simulink model "soc_dvbs2_fpga"  (R2025b)
settings: Solver=FixedStepDiscrete  StartTime=0.0  StopTime=0  RelTol=1e-3
InitFcn:
  | soc_dvbs2_init;
values from neighbouring files (symbols this model uses):
  Rsym = 4e6    (= 4000000)    [soc_dvbs2_init.m]
  soc_dvbs2_txPacketBits = [1 1 0 1 0 1 1 1 0 1 1 1 ... (2972 elements, 2972x1)]    [soc_dvbs2_txPacketBits.mat]
  syncWord = (dec2bin(hex2dec('AC')) - '0').'    [soc_dvbs2_init.m]
  txDataOut = txobj(frameBits(:))    [soc_dvbs2_init.m]
  txFiltCoeff = txobj.pTxFilterCoeff    [soc_dvbs2_init.m]
undefined symbols (not defined in the file or in its folder): Add, coefficientsLog, coefficientsSqrt1, coefficientsSqrt2, dataBits, designMultirateFIR, noisePow, NumBits1, NumBits2, seedsURNG1, seedsURNG2, Shift, Slope1, Slope2, soc_dvbs2_designFIRFilter, txDataOutS1, txDataOutS10, txDataOutS12, txDataOutS13, txDataOutS14, txDataOutS15, txDataOutS16, txDataOutS18, txDataOutS19, txDataOutS2, txDataOutS20, txDataOutS21, txDataOutS22, txDataOutS24, txDataOutS25, txDataOutS26, txDataOutS27, txDataOutS3, txDataOutS4, txDataOutS5, txDataOutS6, txDataOutS7, txDataOutS8, txDataOutS9
libraries: simulink x214, hdlsllib x211, dspsigops x22, dsphdlfiltering2 x8, dsphdlsigops2 x5, commseqgen3 x5, dsphdlmathfun2 x3, hwlogicconnlib x2, whdledac x2, commhdlcrc x2, whdlutilities x1, whdlmod x1
(part 5 of 12)

== system soc_dvbs2_fpga/DVBS2/DVBS2 TxRx/LUT Based Tx/Subsystem1/Subsystem1/txLUT5 ==
  rst : Inport
  enb : Inport  Port=2
  1-D Lookup Table : Lookup_n-D  NumberOfTableDimensions=1  BreakpointsSpecification=Even spacing  BreakpointsForDimension1=0:length(txDataOut)-1  BreakpointsForDimension1FirstPoint=0  Table=fi(DataLUT,1,18,16)  TableDataTypeStr=Inherit: Inherit from 'Table data'  InterpMethod=Flat  InternalRulePriority=Speed  OutDataTypeStr=Inherit: Inherit from 'Table data'  RndMeth=Simplest
  Compare To Constant : simulink/Logic and Bit Operations/Compare To Constant  relop===  const=length(DataLUT) - 2  OutDataTypeStr=boolean
  HDL Counter : hdlsllib/Sources/HDL Counter  CountType=Count limited  CountInit=0  CountStep=1  CountMax=length(DataLUT)-1  CountFromType=Initial value  CountFrom=0  CountResetPort=on  CountLoadPort=off  CountEnbPort=on  CountDirPort=off  CountHitOutputPort=off  CountDataType=Unsigned  CountWordLen=nextpow2(length(DataLUT)-1)  CountFracLen=0  CountSampTime=1
  Out1 : Outport
  endOfLUT : Outport  Port=2
  wires:
  1-D Lookup Table/1 -> Out1/1
  HDL Counter/1 -> Compare To Constant/1, 1-D Lookup Table/1
  enb/1 -> HDL Counter/2
  Compare To Constant/1 -> endOfLUT/1
  rst/1 -> HDL Counter/1

== system soc_dvbs2_fpga/DVBS2/DVBS2 TxRx/LUT Based Tx/Subsystem1/Subsystem1/txLUT6 ==
  rst : Inport
  enb : Inport  Port=2
  1-D Lookup Table : Lookup_n-D  NumberOfTableDimensions=1  BreakpointsSpecification=Even spacing  BreakpointsForDimension1=0:length(txDataOut)-1  BreakpointsForDimension1FirstPoint=0  Table=fi(DataLUT,1,18,16)  TableDataTypeStr=Inherit: Inherit from 'Table data'  InterpMethod=Flat  InternalRulePriority=Speed  OutDataTypeStr=Inherit: Inherit from 'Table data'  RndMeth=Simplest
  Compare To Constant : simulink/Logic and Bit Operations/Compare To Constant  relop===  const=length(DataLUT) - 2  OutDataTypeStr=boolean
  HDL Counter : hdlsllib/Sources/HDL Counter  CountType=Count limited  CountInit=0  CountStep=1  CountMax=length(DataLUT)-1  CountFromType=Initial value  CountFrom=0  CountResetPort=on  CountLoadPort=off  CountEnbPort=on  CountDirPort=off  CountHitOutputPort=off  CountDataType=Unsigned  CountWordLen=nextpow2(length(DataLUT)-1)  CountFracLen=0  CountSampTime=1
  Out1 : Outport
  endOfLUT : Outport  Port=2
  wires:
  rst/1 -> HDL Counter/1
  Compare To Constant/1 -> endOfLUT/1
  enb/1 -> HDL Counter/2
  HDL Counter/1 -> 1-D Lookup Table/1, Compare To Constant/1
  1-D Lookup Table/1 -> Out1/1

== system soc_dvbs2_fpga/DVBS2/DVBS2 TxRx/LUT Based Tx/Subsystem1/Subsystem2/txLUT1 ==
  rst : Inport
  enb : Inport  Port=2
  1-D Lookup Table : Lookup_n-D  NumberOfTableDimensions=1  BreakpointsSpecification=Even spacing  BreakpointsForDimension1=0:length(txDataOut)-1  BreakpointsForDimension1FirstPoint=0  Table=fi(DataLUT,1,18,16)  TableDataTypeStr=Inherit: Inherit from 'Table data'  InterpMethod=Flat  InternalRulePriority=Speed  OutDataTypeStr=Inherit: Inherit from 'Table data'  RndMeth=Simplest
  Compare To Constant : simulink/Logic and Bit Operations/Compare To Constant  relop===  const=length(DataLUT) - 2  OutDataTypeStr=boolean
  HDL Counter : hdlsllib/Sources/HDL Counter  CountType=Count limited  CountInit=0  CountStep=1  CountMax=length(DataLUT)-1  CountFromType=Initial value  CountFrom=0  CountResetPort=on  CountLoadPort=off  CountEnbPort=on  CountDirPort=off  CountHitOutputPort=off  CountDataType=Unsigned  CountWordLen=nextpow2(length(DataLUT)-1)  CountFracLen=0  CountSampTime=1
  Out1 : Outport
  endOfLUT : Outport  Port=2
  wires:
  rst/1 -> HDL Counter/1
  Compare To Constant/1 -> endOfLUT/1
  enb/1 -> HDL Counter/2
  HDL Counter/1 -> 1-D Lookup Table/1, Compare To Constant/1
  1-D Lookup Table/1 -> Out1/1

== system soc_dvbs2_fpga/DVBS2/DVBS2 TxRx/LUT Based Tx/Subsystem1/Subsystem2/txLUT2 ==
  rst : Inport
  enb : Inport  Port=2
  1-D Lookup Table : Lookup_n-D  NumberOfTableDimensions=1  BreakpointsSpecification=Even spacing  BreakpointsForDimension1=0:length(txDataOut)-1  BreakpointsForDimension1FirstPoint=0  Table=fi(DataLUT,1,18,16)  TableDataTypeStr=Inherit: Inherit from 'Table data'  InterpMethod=Flat  InternalRulePriority=Speed  OutDataTypeStr=Inherit: Inherit from 'Table data'  RndMeth=Simplest
  Compare To Constant : simulink/Logic and Bit Operations/Compare To Constant  relop===  const=length(DataLUT) - 2  OutDataTypeStr=boolean
  HDL Counter : hdlsllib/Sources/HDL Counter  CountType=Count limited  CountInit=0  CountStep=1  CountMax=length(DataLUT)-1  CountFromType=Initial value  CountFrom=0  CountResetPort=on  CountLoadPort=off  CountEnbPort=on  CountDirPort=off  CountHitOutputPort=off  CountDataType=Unsigned  CountWordLen=nextpow2(length(DataLUT)-1)  CountFracLen=0  CountSampTime=1
  Out1 : Outport
  endOfLUT : Outport  Port=2
  wires:
  1-D Lookup Table/1 -> Out1/1
  HDL Counter/1 -> Compare To Constant/1, 1-D Lookup Table/1
  enb/1 -> HDL Counter/2
  Compare To Constant/1 -> endOfLUT/1
  rst/1 -> HDL Counter/1

== system soc_dvbs2_fpga/DVBS2/DVBS2 TxRx/LUT Based Tx/Subsystem1/Subsystem2/txLUT3 ==
  rst : Inport
  enb : Inport  Port=2
  1-D Lookup Table : Lookup_n-D  NumberOfTableDimensions=1  BreakpointsSpecification=Even spacing  BreakpointsForDimension1=0:length(txDataOut)-1  BreakpointsForDimension1FirstPoint=0  Table=fi(DataLUT,1,18,16)  TableDataTypeStr=Inherit: Inherit from 'Table data'  InterpMethod=Flat  InternalRulePriority=Speed  OutDataTypeStr=Inherit: Inherit from 'Table data'  RndMeth=Simplest
  Compare To Constant : simulink/Logic and Bit Operations/Compare To Constant  relop===  const=length(DataLUT) - 2  OutDataTypeStr=boolean
  HDL Counter : hdlsllib/Sources/HDL Counter  CountType=Count limited  CountInit=0  CountStep=1  CountMax=length(DataLUT)-1  CountFromType=Initial value  CountFrom=0  CountResetPort=on  CountLoadPort=off  CountEnbPort=on  CountDirPort=off  CountHitOutputPort=off  CountDataType=Unsigned  CountWordLen=nextpow2(length(DataLUT)-1)  CountFracLen=0  CountSampTime=1
  Out1 : Outport
  endOfLUT : Outport  Port=2
  wires:
  1-D Lookup Table/1 -> Out1/1
  HDL Counter/1 -> Compare To Constant/1, 1-D Lookup Table/1
  enb/1 -> HDL Counter/2
  Compare To Constant/1 -> endOfLUT/1
  rst/1 -> HDL Counter/1

== system soc_dvbs2_fpga/DVBS2/DVBS2 TxRx/LUT Based Tx/Subsystem1/Subsystem2/txLUT4 ==
  rst : Inport
  enb : Inport  Port=2
  1-D Lookup Table : Lookup_n-D  NumberOfTableDimensions=1  BreakpointsSpecification=Even spacing  BreakpointsForDimension1=0:length(txDataOut)-1  BreakpointsForDimension1FirstPoint=0  Table=fi(DataLUT,1,18,16)  TableDataTypeStr=Inherit: Inherit from 'Table data'  InterpMethod=Flat  InternalRulePriority=Speed  OutDataTypeStr=Inherit: Inherit from 'Table data'  RndMeth=Simplest
  Compare To Constant : simulink/Logic and Bit Operations/Compare To Constant  relop===  const=length(DataLUT) - 2  OutDataTypeStr=boolean
  HDL Counter : hdlsllib/Sources/HDL Counter  CountType=Count limited  CountInit=0  CountStep=1  CountMax=length(DataLUT)-1  CountFromType=Initial value  CountFrom=0  CountResetPort=on  CountLoadPort=off  CountEnbPort=on  CountDirPort=off  CountHitOutputPort=off  CountDataType=Unsigned  CountWordLen=nextpow2(length(DataLUT)-1)  CountFracLen=0  CountSampTime=1
  Out1 : Outport
  endOfLUT : Outport  Port=2
  wires:
  rst/1 -> HDL Counter/1
  Compare To Constant/1 -> endOfLUT/1
  enb/1 -> HDL Counter/2
  HDL Counter/1 -> 1-D Lookup Table/1, Compare To Constant/1
  1-D Lookup Table/1 -> Out1/1

== system soc_dvbs2_fpga/DVBS2/DVBS2 TxRx/LUT Based Tx/Subsystem1/Subsystem2/txLUT5 ==
  rst : Inport
  enb : Inport  Port=2
  1-D Lookup Table : Lookup_n-D  NumberOfTableDimensions=1  BreakpointsSpecification=Even spacing  BreakpointsForDimension1=0:length(txDataOut)-1  BreakpointsForDimension1FirstPoint=0  Table=fi(DataLUT,1,18,16)  TableDataTypeStr=Inherit: Inherit from 'Table data'  InterpMethod=Flat  InternalRulePriority=Speed  OutDataTypeStr=Inherit: Inherit from 'Table data'  RndMeth=Simplest
  Compare To Constant : simulink/Logic and Bit Operations/Compare To Constant  relop===  const=length(DataLUT) - 2  OutDataTypeStr=boolean
  HDL Counter : hdlsllib/Sources/HDL Counter  CountType=Count limited  CountInit=0  CountStep=1  CountMax=length(DataLUT)-1  CountFromType=Initial value  CountFrom=0  CountResetPort=on  CountLoadPort=off  CountEnbPort=on  CountDirPort=off  CountHitOutputPort=off  CountDataType=Unsigned  CountWordLen=nextpow2(length(DataLUT)-1)  CountFracLen=0  CountSampTime=1
  Out1 : Outport
  endOfLUT : Outport  Port=2
  wires:
  1-D Lookup Table/1 -> Out1/1
  HDL Counter/1 -> Compare To Constant/1, 1-D Lookup Table/1
  enb/1 -> HDL Counter/2
  Compare To Constant/1 -> endOfLUT/1
  rst/1 -> HDL Counter/1

== system soc_dvbs2_fpga/DVBS2/DVBS2 TxRx/LUT Based Tx/Subsystem1/Subsystem2/txLUT6 ==
  rst : Inport
  enb : Inport  Port=2
  1-D Lookup Table : Lookup_n-D  NumberOfTableDimensions=1  BreakpointsSpecification=Even spacing  BreakpointsForDimension1=0:length(txDataOut)-1  BreakpointsForDimension1FirstPoint=0  Table=fi(DataLUT,1,18,16)  TableDataTypeStr=Inherit: Inherit from 'Table data'  InterpMethod=Flat  InternalRulePriority=Speed  OutDataTypeStr=Inherit: Inherit from 'Table data'  RndMeth=Simplest
  Compare To Constant : simulink/Logic and Bit Operations/Compare To Constant  relop===  const=length(DataLUT) - 2  OutDataTypeStr=boolean
  HDL Counter : hdlsllib/Sources/HDL Counter  CountType=Count limited  CountInit=0  CountStep=1  CountMax=length(DataLUT)-1  CountFromType=Initial value  CountFrom=0  CountResetPort=on  CountLoadPort=off  CountEnbPort=on  CountDirPort=off  CountHitOutputPort=off  CountDataType=Unsigned  CountWordLen=nextpow2(length(DataLUT)-1)  CountFracLen=0  CountSampTime=1
  Out1 : Outport
  endOfLUT : Outport  Port=2
  wires:
  rst/1 -> HDL Counter/1
  Compare To Constant/1 -> endOfLUT/1
  enb/1 -> HDL Counter/2
  HDL Counter/1 -> 1-D Lookup Table/1, Compare To Constant/1
  1-D Lookup Table/1 -> Out1/1

== system soc_dvbs2_fpga/DVBS2/DVBS2 TxRx/LUT Based Tx/Subsystem1/Subsystem4/txLUT1 ==
  rst : Inport
  enb : Inport  Port=2
  1-D Lookup Table : Lookup_n-D  NumberOfTableDimensions=1  BreakpointsSpecification=Even spacing  BreakpointsForDimension1=0:length(txDataOut)-1  BreakpointsForDimension1FirstPoint=0  Table=fi(DataLUT,1,18,16)  TableDataTypeStr=Inherit: Inherit from 'Table data'  InterpMethod=Flat  InternalRulePriority=Speed  OutDataTypeStr=Inherit: Inherit from 'Table data'  RndMeth=Simplest
  Compare To Constant : simulink/Logic and Bit Operations/Compare To Constant  relop===  const=length(DataLUT) - 2  OutDataTypeStr=boolean
  HDL Counter : hdlsllib/Sources/HDL Counter  CountType=Count limited  CountInit=0  CountStep=1  CountMax=length(DataLUT)-1  CountFromType=Initial value  CountFrom=0  CountResetPort=on  CountLoadPort=off  CountEnbPort=on  CountDirPort=off  CountHitOutputPort=off  CountDataType=Unsigned  CountWordLen=nextpow2(length(DataLUT)-1)  CountFracLen=0  CountSampTime=1
  Out1 : Outport
  endOfLUT : Outport  Port=2
  wires:
  1-D Lookup Table/1 -> Out1/1
  HDL Counter/1 -> Compare To Constant/1, 1-D Lookup Table/1
  enb/1 -> HDL Counter/2
  Compare To Constant/1 -> endOfLUT/1
  rst/1 -> HDL Counter/1

== system soc_dvbs2_fpga/DVBS2/DVBS2 TxRx/LUT Based Tx/Subsystem1/Subsystem4/txLUT2 ==
  rst : Inport
  enb : Inport  Port=2
  1-D Lookup Table : Lookup_n-D  NumberOfTableDimensions=1  BreakpointsSpecification=Even spacing  BreakpointsForDimension1=0:length(txDataOut)-1  BreakpointsForDimension1FirstPoint=0  Table=fi(DataLUT,1,18,16)  TableDataTypeStr=Inherit: Inherit from 'Table data'  InterpMethod=Flat  InternalRulePriority=Speed  OutDataTypeStr=Inherit: Inherit from 'Table data'  RndMeth=Simplest
  Compare To Constant : simulink/Logic and Bit Operations/Compare To Constant  relop===  const=length(DataLUT) - 2  OutDataTypeStr=boolean
  HDL Counter : hdlsllib/Sources/HDL Counter  CountType=Count limited  CountInit=0  CountStep=1  CountMax=length(DataLUT)-1  CountFromType=Initial value  CountFrom=0  CountResetPort=on  CountLoadPort=off  CountEnbPort=on  CountDirPort=off  CountHitOutputPort=off  CountDataType=Unsigned  CountWordLen=nextpow2(length(DataLUT)-1)  CountFracLen=0  CountSampTime=1
  Out1 : Outport
  endOfLUT : Outport  Port=2
  wires:
  rst/1 -> HDL Counter/1
  Compare To Constant/1 -> endOfLUT/1
  enb/1 -> HDL Counter/2
  HDL Counter/1 -> 1-D Lookup Table/1, Compare To Constant/1
  1-D Lookup Table/1 -> Out1/1

== system soc_dvbs2_fpga/DVBS2/DVBS2 TxRx/LUT Based Tx/Subsystem1/Subsystem4/txLUT3 ==
  rst : Inport
  enb : Inport  Port=2
  1-D Lookup Table : Lookup_n-D  NumberOfTableDimensions=1  BreakpointsSpecification=Even spacing  BreakpointsForDimension1=0:length(txDataOut)-1  BreakpointsForDimension1FirstPoint=0  Table=fi(DataLUT,1,18,16)  TableDataTypeStr=Inherit: Inherit from 'Table data'  InterpMethod=Flat  InternalRulePriority=Speed  OutDataTypeStr=Inherit: Inherit from 'Table data'  RndMeth=Simplest
  Compare To Constant : simulink/Logic and Bit Operations/Compare To Constant  relop===  const=length(DataLUT) - 2  OutDataTypeStr=boolean
  HDL Counter : hdlsllib/Sources/HDL Counter  CountType=Count limited  CountInit=0  CountStep=1  CountMax=length(DataLUT)-1  CountFromType=Initial value  CountFrom=0  CountResetPort=on  CountLoadPort=off  CountEnbPort=on  CountDirPort=off  CountHitOutputPort=off  CountDataType=Unsigned  CountWordLen=nextpow2(length(DataLUT)-1)  CountFracLen=0  CountSampTime=1
  Out1 : Outport
  endOfLUT : Outport  Port=2
  wires:
  rst/1 -> HDL Counter/1
  Compare To Constant/1 -> endOfLUT/1
  enb/1 -> HDL Counter/2
  HDL Counter/1 -> 1-D Lookup Table/1, Compare To Constant/1
  1-D Lookup Table/1 -> Out1/1

== system soc_dvbs2_fpga/DVBS2/DVBS2 TxRx/LUT Based Tx/Subsystem1/Subsystem4/txLUT4 ==
  rst : Inport
  enb : Inport  Port=2
  1-D Lookup Table : Lookup_n-D  NumberOfTableDimensions=1  BreakpointsSpecification=Even spacing  BreakpointsForDimension1=0:length(txDataOut)-1  BreakpointsForDimension1FirstPoint=0  Table=fi(DataLUT,1,18,16)  TableDataTypeStr=Inherit: Inherit from 'Table data'  InterpMethod=Flat  InternalRulePriority=Speed  OutDataTypeStr=Inherit: Inherit from 'Table data'  RndMeth=Simplest
  Compare To Constant : simulink/Logic and Bit Operations/Compare To Constant  relop===  const=length(DataLUT) - 2  OutDataTypeStr=boolean
  HDL Counter : hdlsllib/Sources/HDL Counter  CountType=Count limited  CountInit=0  CountStep=1  CountMax=length(DataLUT)-1  CountFromType=Initial value  CountFrom=0  CountResetPort=on  CountLoadPort=off  CountEnbPort=on  CountDirPort=off  CountHitOutputPort=off  CountDataType=Unsigned  CountWordLen=nextpow2(length(DataLUT)-1)  CountFracLen=0  CountSampTime=1
  Out1 : Outport
  endOfLUT : Outport  Port=2
  wires:
  1-D Lookup Table/1 -> Out1/1
  HDL Counter/1 -> Compare To Constant/1, 1-D Lookup Table/1
  enb/1 -> HDL Counter/2
  Compare To Constant/1 -> endOfLUT/1
  rst/1 -> HDL Counter/1

== system soc_dvbs2_fpga/DVBS2/DVBS2 TxRx/LUT Based Tx/Subsystem1/Subsystem4/txLUT5 ==
  rst : Inport
  enb : Inport  Port=2
  1-D Lookup Table : Lookup_n-D  NumberOfTableDimensions=1  BreakpointsSpecification=Even spacing  BreakpointsForDimension1=0:length(txDataOut)-1  BreakpointsForDimension1FirstPoint=0  Table=fi(DataLUT,1,18,16)  TableDataTypeStr=Inherit: Inherit from 'Table data'  InterpMethod=Flat  InternalRulePriority=Speed  OutDataTypeStr=Inherit: Inherit from 'Table data'  RndMeth=Simplest
  Compare To Constant : simulink/Logic and Bit Operations/Compare To Constant  relop===  const=length(DataLUT) - 2  OutDataTypeStr=boolean
  HDL Counter : hdlsllib/Sources/HDL Counter  CountType=Count limited  CountInit=0  CountStep=1  CountMax=length(DataLUT)-1  CountFromType=Initial value  CountFrom=0  CountResetPort=on  CountLoadPort=off  CountEnbPort=on  CountDirPort=off  CountHitOutputPort=off  CountDataType=Unsigned  CountWordLen=nextpow2(length(DataLUT)-1)  CountFracLen=0  CountSampTime=1
  Out1 : Outport
  endOfLUT : Outport  Port=2
  wires:
  rst/1 -> HDL Counter/1
  Compare To Constant/1 -> endOfLUT/1
  enb/1 -> HDL Counter/2
  HDL Counter/1 -> 1-D Lookup Table/1, Compare To Constant/1
  1-D Lookup Table/1 -> Out1/1

== system soc_dvbs2_fpga/DVBS2/DVBS2 TxRx/LUT Based Tx/Subsystem1/Subsystem4/txLUT6 ==
  rst : Inport
  enb : Inport  Port=2
  1-D Lookup Table : Lookup_n-D  NumberOfTableDimensions=1  BreakpointsSpecification=Even spacing  BreakpointsForDimension1=0:length(txDataOut)-1  BreakpointsForDimension1FirstPoint=0  Table=fi(DataLUT,1,18,16)  TableDataTypeStr=Inherit: Inherit from 'Table data'  InterpMethod=Flat  InternalRulePriority=Speed  OutDataTypeStr=Inherit: Inherit from 'Table data'  RndMeth=Simplest
  Compare To Constant : simulink/Logic and Bit Operations/Compare To Constant  relop===  const=length(DataLUT) - 2  OutDataTypeStr=boolean
  HDL Counter : hdlsllib/Sources/HDL Counter  CountType=Count limited  CountInit=0  CountStep=1  CountMax=length(DataLUT)-1  CountFromType=Initial value  CountFrom=0  CountResetPort=on  CountLoadPort=off  CountEnbPort=on  CountDirPort=off  CountHitOutputPort=off  CountDataType=Unsigned  CountWordLen=nextpow2(length(DataLUT)-1)  CountFracLen=0  CountSampTime=1
  Out1 : Outport
  endOfLUT : Outport  Port=2
  wires:
  1-D Lookup Table/1 -> Out1/1
  HDL Counter/1 -> Compare To Constant/1, 1-D Lookup Table/1
  enb/1 -> HDL Counter/2
  Compare To Constant/1 -> endOfLUT/1
  rst/1 -> HDL Counter/1

== system soc_dvbs2_fpga/DVBS2/DVBS2 TxRx/Channel/AWGN Generator/Unit Variance Gaussian Noise/SqrtImplementation/SqrtEval ==
  u : Inport
  FunctionEvaluation : Subsystem
  RangeReconstruction : Subsystem
  RangeReduction : Subsystem
  f : Outport
  wires:
  FunctionEvaluation/1(y_f) -> RangeReconstruction/1(y_f)
  u/1 -> RangeReduction/1(u)
  RangeReconstruction/1(f) -> f/1
  RangeReduction/1(x_f) -> FunctionEvaluation/1(x_f)
  RangeReduction/2(pass) -> FunctionEvaluation/2(passIn)
  RangeReduction/3(exp_f) -> FunctionEvaluation/3(exp_fIn)
  FunctionEvaluation/2(passOut) -> RangeReconstruction/2(pass)
  FunctionEvaluation/3(exp_fOut) -> RangeReconstruction/3(exp_f)

== system soc_dvbs2_fpga/DVBS2/DVBS2 TxRx/Channel/AWGN Generator/Unit Variance Gaussian Noise/TausUniformRandGen/ConcatandExtract ==
  a : Inport
  b : Inport  Port=2
  Bit Concat : hdlsllib/Logic and Bit Operations/Bit Concat  numInputs=2
  Bitwise Operator : simulink/Logic and Bit Operations/Bitwise Operator  logicop=AND  UseBitMask=on  BitMask=bin2dec('00000000000000001111111111111111')  BitMaskRealWorld=Stored Integer
  Data Type Conversion : DataTypeConversion  OutDataTypeStr=uint16  SaturateOnIntegerOverflow=off  RndMeth=Floor
  Data Type Conversion2 : DataTypeConversion  OutDataTypeStr=fixdt(0,16,0)  SaturateOnIntegerOverflow=off  RndMeth=Floor
  Shift Arithmetic : ArithShift  BinPtShiftNumber=-16
  Shift Arithmetic1 : ArithShift  BinPtShiftNumber=-48
  Shift Arithmetic2 : ArithShift  BitShiftNumber=16  BitShiftDirection=Right
  u0(48,48) : Outport
  u1(16,16) : Outport  Port=2
  wires:
  Shift Arithmetic1/1 -> u0(48,48)/1  "u0(48,48)"
  Bit Concat/1 -> Shift Arithmetic1/1  "u0(48,0)"
  b/1 -> Bitwise Operator/1, Shift Arithmetic2/1
  Shift Arithmetic2/1 -> Data Type Conversion/1
  Bitwise Operator/1 -> Data Type Conversion2/1
  Data Type Conversion/1 -> Bit Concat/2
  a/1 -> Bit Concat/1
  Data Type Conversion2/1 -> Shift Arithmetic/1
  Shift Arithmetic/1 -> u1(16,16)/1  "u0(16,16)"

== system soc_dvbs2_fpga/DVBS2/DVBS2 TxRx/Channel/AWGN Generator/Unit Variance Gaussian Noise/TausUniformRandGen/TausURNG1 ==
  note: S0
  note: S1
  note: S1
  Bit Shift : hdlsllib/Logic and Bit Operations/Bit Shift  mode=Shift Left Logical  N=13
  Bit Shift1 : hdlsllib/Logic and Bit Operations/Bit Shift  mode=Shift Right Logical  N=19
  Bit Shift2 : hdlsllib/Logic and Bit Operations/Bit Shift  mode=Shift Left Logical  N=12
  Bit Shift3 : hdlsllib/Logic and Bit Operations/Bit Shift  mode=Shift Left Logical  N=2
  Bit Shift4 : hdlsllib/Logic and Bit Operations/Bit Shift  mode=Shift Left Logical  N=4
  Bit Shift5 : hdlsllib/Logic and Bit Operations/Bit Shift  mode=Shift Right Logical  N=25
  Bit Shift6 : hdlsllib/Logic and Bit Operations/Bit Shift  mode=Shift Left Logical  N=3
  Bit Shift7 : hdlsllib/Logic and Bit Operations/Bit Shift  mode=Shift Left Logical  N=17
  Bit Shift8 : hdlsllib/Logic and Bit Operations/Bit Shift  mode=Shift Right Logical  N=11
  Bitwise Operator{,2..3,5..6,8} (6 alike) : simulink/Logic and Bit Operations/Bitwise Operator  logicop=XOR  UseBitMask=off  NumInputPorts=2  BitMask=bin2dec('11011001')  BitMaskRealWorld=Stored Integer
  Bitwise Operator1 : simulink/Logic and Bit Operations/Bitwise Operator  logicop=AND  UseBitMask=on  BitMask=fi(4294967294, 0, 32, 0);  BitMaskRealWorld=Stored Integer
  Bitwise Operator4 : simulink/Logic and Bit Operations/Bitwise Operator  logicop=AND  UseBitMask=on  BitMask=fi(4294967288, 0, 32, 0);  BitMaskRealWorld=Stored Integer
  Bitwise Operator7 : simulink/Logic and Bit Operations/Bitwise Operator  logicop=AND  UseBitMask=on  BitMask=fi(4294967280, 0, 32, 0);  BitMaskRealWorld=Stored Integer
  Bitwise Operator9 : simulink/Logic and Bit Operations/Bitwise Operator  logicop=XOR  UseBitMask=off  NumInputPorts=3  BitMask=bin2dec('11011001')  BitMaskRealWorld=Stored Integer
  Data Type Conversion : DataTypeConversion  OutDataTypeStr=uint32  SaturateOnIntegerOverflow=off  RndMeth=Floor
  Data Type Conversion1 : DataTypeConversion  OutDataTypeStr=uint32  SaturateOnIntegerOverflow=off  RndMeth=Floor
  Data Type Conversion2 : DataTypeConversion  OutDataTypeStr=uint32  SaturateOnIntegerOverflow=off  RndMeth=Floor
  Delay : Delay  DelayLength=1  InitialCondition=seedsURNG1(1)
  Delay1 : Delay  DelayLength=1  InitialCondition=seedsURNG1(2)
  Delay2 : Delay  DelayLength=1  InitialCondition=seedsURNG1(3)
  a : Outport
  wires:
  Bit Shift1/1 -> Bitwise Operator2/1
  Bitwise Operator2/1 -> Bitwise Operator9/1, Delay/1
  Bit Shift/1 -> Bitwise Operator/1
  Bitwise Operator/1 -> Bit Shift1/1
  Bitwise Operator1/1 -> Bit Shift2/1
  Bit Shift2/1 -> Bitwise Operator2/2
  Bit Shift4/1 -> Bitwise Operator5/2
  Bit Shift3/1 -> Bitwise Operator3/1
  Bitwise Operator4/1 -> Bit Shift4/1
  Bitwise Operator5/1 -> Delay1/1, Bitwise Operator9/2
  Bitwise Operator3/1 -> Bit Shift5/1
  Bit Shift5/1 -> Bitwise Operator5/1
  Bitwise Operator7/1 -> Bit Shift7/1
  Bitwise Operator8/1 -> Bitwise Operator9/3, Delay2/1
  Bit Shift6/1 -> Bitwise Operator6/1
  Bit Shift7/1 -> Bitwise Operator8/2
  Bitwise Operator6/1 -> Bit Shift8/1
  Bit Shift8/1 -> Bitwise Operator8/1
  Delay/1 -> Data Type Conversion/1
  Delay1/1 -> Data Type Conversion1/1
  Delay2/1 -> Data Type Conversion2/1
  Bitwise Operator9/1 -> a/1
  Data Type Conversion/1 -> Bit Shift/1, Bitwise Operator1/1, Bitwise Operator/2
  Data Type Conversion1/1 -> Bit Shift3/1, Bitwise Operator3/2, Bitwise Operator4/1
  Data Type Conversion2/1 -> Bit Shift6/1, Bitwise Operator7/1, Bitwise Operator6/2

== system soc_dvbs2_fpga/DVBS2/DVBS2 TxRx/Channel/AWGN Generator/Unit Variance Gaussian Noise/TausUniformRandGen/TausURNG2 ==
  note: S0
  note: S1
  note: S1
  Bit Shift : hdlsllib/Logic and Bit Operations/Bit Shift  mode=Shift Left Logical  N=13
  Bit Shift1 : hdlsllib/Logic and Bit Operations/Bit Shift  mode=Shift Right Logical  N=19
  Bit Shift2 : hdlsllib/Logic and Bit Operations/Bit Shift  mode=Shift Left Logical  N=12
  Bit Shift3 : hdlsllib/Logic and Bit Operations/Bit Shift  mode=Shift Left Logical  N=2
  Bit Shift4 : hdlsllib/Logic and Bit Operations/Bit Shift  mode=Shift Left Logical  N=4
  Bit Shift5 : hdlsllib/Logic and Bit Operations/Bit Shift  mode=Shift Right Logical  N=25
  Bit Shift6 : hdlsllib/Logic and Bit Operations/Bit Shift  mode=Shift Left Logical  N=3
  Bit Shift7 : hdlsllib/Logic and Bit Operations/Bit Shift  mode=Shift Left Logical  N=17
  Bit Shift8 : hdlsllib/Logic and Bit Operations/Bit Shift  mode=Shift Right Logical  N=11
  Bitwise Operator{,2..3,5..6,8} (6 alike) : simulink/Logic and Bit Operations/Bitwise Operator  logicop=XOR  UseBitMask=off  NumInputPorts=2  BitMask=bin2dec('11011001')  BitMaskRealWorld=Stored Integer
  Bitwise Operator1 : simulink/Logic and Bit Operations/Bitwise Operator  logicop=AND  UseBitMask=on  BitMask=fi(4294967294, 0, 32, 0);  BitMaskRealWorld=Stored Integer
  Bitwise Operator4 : simulink/Logic and Bit Operations/Bitwise Operator  logicop=AND  UseBitMask=on  BitMask=fi(4294967288, 0, 32, 0);  BitMaskRealWorld=Stored Integer
  Bitwise Operator7 : simulink/Logic and Bit Operations/Bitwise Operator  logicop=AND  UseBitMask=on  BitMask=fi(4294967280, 0, 32, 0);  BitMaskRealWorld=Stored Integer
  Bitwise Operator9 : simulink/Logic and Bit Operations/Bitwise Operator  logicop=XOR  UseBitMask=off  NumInputPorts=3  BitMask=bin2dec('11011001')  BitMaskRealWorld=Stored Integer
  Data Type Conversion : DataTypeConversion  OutDataTypeStr=uint32  SaturateOnIntegerOverflow=off  RndMeth=Floor
  Data Type Conversion1 : DataTypeConversion  OutDataTypeStr=uint32  SaturateOnIntegerOverflow=off  RndMeth=Floor
  Data Type Conversion2 : DataTypeConversion  OutDataTypeStr=uint32  SaturateOnIntegerOverflow=off  RndMeth=Floor
  Delay : Delay  DelayLength=1  InitialCondition=seedsURNG2(1)
  Delay1 : Delay  DelayLength=1  InitialCondition=seedsURNG2(2)
  Delay2 : Delay  DelayLength=1  InitialCondition=seedsURNG2(3)
  b : Outport
  wires:
  Bit Shift1/1 -> Bitwise Operator2/1
  Bitwise Operator2/1 -> Bitwise Operator9/1, Delay/1
  Bit Shift/1 -> Bitwise Operator/1
  Bitwise Operator/1 -> Bit Shift1/1
  Bitwise Operator1/1 -> Bit Shift2/1
  Bit Shift2/1 -> Bitwise Operator2/2
  Bit Shift4/1 -> Bitwise Operator5/2
  Bit Shift3/1 -> Bitwise Operator3/1
  Bitwise Operator4/1 -> Bit Shift4/1
  Bitwise Operator5/1 -> Delay1/1, Bitwise Operator9/2
  Bitwise Operator3/1 -> Bit Shift5/1
  Bit Shift5/1 -> Bitwise Operator5/1
  Bitwise Operator7/1 -> Bit Shift7/1
  Bitwise Operator8/1 -> Bitwise Operator9/3, Delay2/1
  Bit Shift6/1 -> Bitwise Operator6/1
  Bit Shift7/1 -> Bitwise Operator8/2
  Bitwise Operator6/1 -> Bit Shift8/1
  Bit Shift8/1 -> Bitwise Operator8/1
  Delay/1 -> Data Type Conversion/1
  Delay1/1 -> Data Type Conversion1/1
  Delay2/1 -> Data Type Conversion2/1
  Bitwise Operator9/1 -> b/1
  Data Type Conversion/1 -> Bit Shift/1, Bitwise Operator1/1, Bitwise Operator/2
  Data Type Conversion1/1 -> Bit Shift3/1, Bitwise Operator4/1, Bitwise Operator3/2
  Data Type Conversion2/1 -> Bit Shift6/1, Bitwise Operator7/1, Bitwise Operator6/2

== system soc_dvbs2_fpga/DVBS2/DVBS2 TxRx/Channel/AWGN Generator/Unit Variance Gaussian Noise/logImplementation/log ==
  u0(48,48) : Inport
  FunctionEvaluation : Subsystem
  RangeReconstruction : Subsystem
  RangeReduction : Subsystem
  e : Outport  VectorParamsAs1DForOutWhenUnconnected=off
  wires:
  u0(48,48)/1 -> RangeReduction/1(x)
  FunctionEvaluation/1(y_e) -> RangeReconstruction/1(y_e)
  RangeReconstruction/1(e) -> e/1
  RangeReduction/1(x_e) -> FunctionEvaluation/1(x_e)
  RangeReduction/2(exp_e) -> FunctionEvaluation/2(exp_eIn)
  FunctionEvaluation/2(exp_eOut) -> RangeReconstruction/2(exp_e)

== system soc_dvbs2_fpga/DVBS2/DVBS2 TxRx/DVB-S2 HDL Receiver/Demod Deinterleave and FECDecode/DVBS2 HDL Deinterleaver/RAM/Single RAM Using Two RAMs ==
  wr_din : Inport
  wr_addr : Inport  Port=2
  wr_en : Inport  Port=3
  rd_addr : Inport  Port=4
  Delay : Delay  DelayLength=1
  Extract Bits : simulink/Logic and Bit Operations/Extract Bits  bitsToExtract=Range of bits  numBits=8  bitIdxRange=[0 15]  outScalingMode=Treat bit field as an integer
  Extract Bits1 : simulink/Logic and Bit Operations/Extract Bits  bitsToExtract=Range of bits  numBits=8  bitIdxRange=16  outScalingMode=Treat bit field as an integer
  Extract Bits2 : simulink/Logic and Bit Operations/Extract Bits  bitsToExtract=Range of bits  numBits=8  bitIdxRange=[0 15]  outScalingMode=Treat bit field as an integer
  Extract Bits3 : simulink/Logic and Bit Operations/Extract Bits  bitsToExtract=Range of bits  numBits=8  bitIdxRange=16  outScalingMode=Treat bit field as an integer
  Logical Operator1 : Logic  Operator=NOT  AllPortsSameDT=off  OutDataTypeStr=boolean
  Logical Operator2 : Logic  AllPortsSameDT=off  OutDataTypeStr=boolean
  Logical Operator3 : Logic  AllPortsSameDT=off  OutDataTypeStr=boolean
  Multiport Switch : MultiPortSwitch  DataPortOrder=Zero-based contiguous  Inputs=2  zeroidx=on  SaturateOnIntegerOverflow=off  InputSameDT=off
  Simple Dual Port RAM : hdlsllib/HDL RAMs/Simple Dual Port RAM  ram_size=nextpow2(ConfigRx.RAMCapacity/2)
  Simple Dual Port RAM1 : hdlsllib/HDL RAMs/Simple Dual Port RAM  ram_size=nextpow2(ConfigRx.RAMCapacity/2)
  rd_dout : Outport
  wires:
  wr_addr/1 -> Extract Bits/1, Extract Bits1/1
  wr_en/1 -> Logical Operator3/2, Logical Operator2/2
  rd_addr/1 -> Extract Bits2/1, Extract Bits3/1
  wr_din/1 -> Simple Dual Port RAM1/1, Simple Dual Port RAM/1
  Simple Dual Port RAM/1 -> Multiport Switch/2
  Extract Bits/1 -> Simple Dual Port RAM/2, Simple Dual Port RAM1/2
  Extract Bits1/1 -> Logical Operator1/1, Logical Operator2/1
  Logical Operator1/1 -> Logical Operator3/1
  Logical Operator3/1 -> Simple Dual Port RAM/3
  Logical Operator2/1 -> Simple Dual Port RAM1/3
  Extract Bits2/1 -> Simple Dual Port RAM/4, Simple Dual Port RAM1/4
  Extract Bits3/1 -> Delay/1
  Simple Dual Port RAM1/1 -> Multiport Switch/3
  Multiport Switch/1 -> rd_dout/1
  Delay/1 -> Multiport Switch/1

== system soc_dvbs2_fpga/DVBS2/DVBS2 TxRx/DVB-S2 HDL Receiver/Demod Deinterleave and FECDecode/DVBS2 HDL Deinterleaver/RAM/Wrap Address ==
  u : Inport
  Add : Sum  Inputs=+-  OutDataTypeStr=Inherit: Same as first input
  Compare To Constant : simulink/Logic and Bit Operations/Compare To Constant  relop=>=  const=ConfigRx.RAMCapacity  OutDataTypeStr=boolean
  Constant : Constant  Value=ConfigRx.RAMCapacity  OutDataTypeStr=Inherit: Inherit via back propagation  SampleTime=Tsamp
  Constant1 : Constant  Value=0  OutDataTypeStr=Inherit: Inherit via back propagation  SampleTime=Tsamp
  Data Type Duplicate : DataTypeDuplicate
  Data Type Duplicate1 : DataTypeDuplicate
  Data Type Conversion : DataTypeConversion  OutDataTypeStr=fixdt(0,nextpow2(ConfigRx.RAMCapacity),0)  SaturateOnIntegerOverflow=off  RndMeth=Floor
  Switch : Switch  Criteria=u2 ~= 0  SaturateOnIntegerOverflow=off  InputSameDT=off
  Switch1 : Switch  Criteria=u2 ~= 0  SaturateOnIntegerOverflow=off  InputSameDT=off
  y : Outport
  wires:
  Constant1/1 -> Switch1/3, Data Type Duplicate1/2
  Switch1/1 -> Add/2
  Data Type Conversion/1 -> y/1
  Constant/1 -> Data Type Duplicate/2, Data Type Duplicate1/1, Switch1/1
  Add/1 -> Switch/1
  Compare To Constant/1 -> Switch/2, Switch1/2
  Switch/1 -> Data Type Conversion/1
  u/1 -> Compare To Constant/1, Add/1, Data Type Duplicate/1, Switch/3

== system soc_dvbs2_fpga/DVBS2/DVBS2 TxRx/DVB-S2 HDL Receiver/Demod Deinterleave and FECDecode/DVBS2 HDL Deinterleaver/RAM Address Generator/Generate and Add Read Base Address ==
  readAddrIn : Inport
  readValidIn : Inport  Port=2
  startIn : Inport  Port=3
  endIn : Inport  Port=4
  Add : Sum  Inputs=|++
  Delay{,1,3..4,18} (5 alike) : Delay  DelayLength=1
  Delay{5..9,11,13..16,19..20} (12 alike) : Delay
  Gain : Gain  Gain=ConfigRx.ShortFrameLen  ParamDataTypeStr=fixdt(0,nextpow2(16200),0)
  HDL Counter : hdlsllib/Sources/HDL Counter  CountType=Count limited  CountInit=0  CountStep=1  CountMax=(ConfigRx.RAMCapacity/ConfigRx.ShortFrameLen) - 1  CountFromType=Initial value  CountFrom=0  CountResetPort=off  CountLoadPort=off  CountEnbPort=on  CountDirPort=off  CountHitOutputPort=off  CountDataType=Unsigned  CountWordLen=nextpow2((ConfigRx.RAMCapacity/ConfigRx.ShortFrameLen) - 1)  CountFracLen=0  CountSampTime=1
  Indicate End of Every ShortFrame Length Samples : Subsystem
  Logical Operator : Logic  AllPortsSameDT=off  OutDataTypeStr=boolean
  No HDL Read Address Debug Scope : Subsystem
      settings: PortSchema="{\"entries\":[{\"content\":{\"sides\":[{\"content\":{\"connectorIds\":[]},\"type\":\"ConnectorPlacement.EquallySpacedRectSide\",\"uuid\":\"46203939-3922-41f1-8ac4-248045cc482a\"},{\"content\":{\"connectorIds\":[],\"side\":\"RIGHT\"},\"type\":\"ConnectorPlacement.EquallySpacedRectSide\",\"uuid\":\"e2b32fd8-ba43-4add-9433-a5e10ef1a6cd\"},{\"content\":{\"connectorIds\":[],\"side\":\"TOP\"},\"type\":\"ConnectorPlacement.EquallySpacedRectSide\",\"uuid\":\"bfa555b4-8f13-4832-b51a-da5c9f2f7d4d\"},{\"content\":{\"connectorIds\":[\"In1\",\"In2\",\"In3\",\"In4\"],\"side\":\"BOTTOM\"},\"type\":\"ConnectorPlacement.EquallySpacedRectSide\",\"uuid\":\"1df13975-2c0e-47d4-aefc-7a99adf3a0bb\"}]},\"type\":\"ConnectorPlacement.EquallySpacedConnector\",\"uuid\":\"18a89938-2c8d-49b5-957c-22a1a70f8f87\"}],\"packageUris\":[\"http://schema.mathworks.com/mf0/Connector/R2020b\"],\"version\":\"1.0\"}"
  Unit Delay Enabled Synchronous3 : hdlsllib/Discrete/Unit Delay Enabled Synchronous  InitialCondition=0.0  SampleTime=-1
  readAddrOut : Outport
  readValidOut : Outport  Port=2
  readStartOut : Outport  Port=3
  readEndOut : Outport  Port=4
  wires:
  Delay20/1 -> readStartOut/1
  Delay19/1 -> Delay20/1
  Delay18/1 -> Delay19/1
  startIn/1 -> Delay18/1
  Delay16/1 -> readValidOut/1
  Delay15/1 -> No HDL Read Address Debug Scope/3(offsetAddr), Add/1
  Delay14/1 -> Delay16/1
  Delay13/1 -> Delay15/1
  Delay11/1 -> readEndOut/1
  Delay9/1 -> Delay11/1
  Delay8/1 -> Unit Delay Enabled Synchronous3/2
  Delay7/1 -> No HDL Read Address Debug Scope/2(captureBaseAddrIdx), Delay8/1
  Delay6/1 -> Unit Delay Enabled Synchronous3/1
  Delay5/1 -> Gain/1
  Delay4/1 -> Delay14/1
  Delay3/1 -> Delay13/1
  Delay1/1 -> Delay9/1
  Delay/1 -> Delay7/1
  endIn/1 -> Delay/1, Delay1/1
  readValidIn/1 -> Delay4/1, Logical Operator/2
  Add/1 -> No HDL Read Address Debug Scope/4(basePlusOffsetAddr), readAddrOut/1
  Unit Delay Enabled Synchronous3/1 -> Add/2
  Logical Operator/1 -> HDL Counter/1
  HDL Counter/1 -> No HDL Read Address Debug Scope/1(baseAddrIdx), Delay5/1
  readAddrIn/1 -> Delay3/1, Indicate End of Every ShortFrame Length Samples/1(readAddr)
  Indicate End of Every ShortFrame Length Samples/1(endIndicate) -> Logical Operator/1
  Gain/1 -> Delay6/1

== system soc_dvbs2_fpga/DVBS2/DVBS2 TxRx/DVB-S2 HDL Receiver/Demod Deinterleave and FECDecode/DVBS2 HDL Deinterleaver/RAM Address Generator/Parameter Store FIFO ==
  writeVal : Inport
  modIdxOut : Inport  Port=2
  codIdxOut : Inport  Port=3
  fecFrameOut : Inport  Port=4
  readVal : Inport  Port=5
  Delay1 : Delay  DelayLength=3
  Delay{6,8..14,21..23,25} (12 alike) : Delay  DelayLength=1
  Delay{3..5,7,15..20,24,26,28..29} (14 alike) : Delay
  Delay2 : Delay  DelayLength=3
  Delay27 : Delay  DelayLength=5
  Fec Frame FIFO : hdlsllib/HDL RAMs/Simple Dual Port RAM  ram_size=log2(8)
  ReadVal Address : hdlsllib/Sources/HDL Counter  CountType=Count limited  CountInit=0  CountStep=1  CountMax=7  CountFromType=Initial value  CountFrom=0  CountResetPort=off  CountLoadPort=off  CountEnbPort=on  CountDirPort=off  CountHitOutputPort=off  CountDataType=Unsigned  CountWordLen=3  CountFracLen=0  CountSampTime=1
  Simple Dual Port RAM2 : hdlsllib/HDL RAMs/Simple Dual Port RAM  ram_size=log2(8)
  WriteVal Address : hdlsllib/Sources/HDL Counter  CountType=Count limited  CountInit=0  CountStep=1  CountMax=7  CountFromType=Initial value  CountFrom=0  CountResetPort=off  CountLoadPort=off  CountEnbPort=on  CountDirPort=off  CountHitOutputPort=off  CountDataType=Unsigned  CountWordLen=3  CountFracLen=0  CountSampTime=1
  cod Idx FIFO : hdlsllib/HDL RAMs/Simple Dual Port RAM  ram_size=log2(8)
  codIdx : Outport
  fecframe : Outport  Port=2
  modIdx : Outport  Port=3
  wires:
  Delay20/1 -> Fec Frame FIFO/4
  Delay19/1 -> Fec Frame FIFO/3
  Delay18/1 -> Fec Frame FIFO/2
  Delay17/1 -> Fec Frame FIFO/1
  Delay16/1 -> cod Idx FIFO/4
  Delay15/1 -> cod Idx FIFO/3
  Delay14/1 -> Delay20/1
  Delay13/1 -> Delay19/1
  Delay12/1 -> Delay18/1
  Delay11/1 -> Delay17/1
  Delay10/1 -> Delay16/1
  Delay9/1 -> Delay15/1
  Delay8/1 -> Delay7/1
  Delay6/1 -> Delay5/1
  Delay7/1 -> cod Idx FIFO/2
  Delay5/1 -> cod Idx FIFO/1
  Delay4/1 -> Delay2/1
  Delay3/1 -> Delay1/1
  Delay2/1 -> fecframe/1
  Delay1/1 -> codIdx/1
  Fec Frame FIFO/1 -> Delay4/1
  fecFrameOut/1 -> Delay11/1
  cod Idx FIFO/1 -> Delay3/1
  codIdxOut/1 -> Delay6/1
  readVal/1 -> ReadVal Address/1
  Simple Dual Port RAM2/1 -> Delay27/1
  modIdxOut/1 -> Delay22/1
  WriteVal Address/1 -> Delay21/1, Delay12/1, Delay8/1
  writeVal/1 -> Delay9/1, WriteVal Address/1, Delay23/1, Delay13/1
  ReadVal Address/1 -> Delay25/1, Delay14/1, Delay10/1
  Delay27/1 -> modIdx/1
  Delay22/1 -> Delay24/1
  Delay21/1 -> Delay26/1
  Delay23/1 -> Delay28/1
  Delay25/1 -> Delay29/1
  Delay24/1 -> Simple Dual Port RAM2/1
  Delay26/1 -> Simple Dual Port RAM2/2
  Delay28/1 -> Simple Dual Port RAM2/3
  Delay29/1 -> Simple Dual Port RAM2/4

== system soc_dvbs2_fpga/DVBS2/DVBS2 TxRx/DVB-S2 HDL Receiver/Demod Deinterleave and FECDecode/DVBS2 HDL Deinterleaver/RAM Address Generator/Read Offset Address ==
  maxR : Inport
  maxC : Inport  Port=2
  modcodIs12 : Inport  Port=3
  wrAddr : Inport  Port=4
  wrEnb : Inport  Port=5
  Compute Read Offset Address : Subsystem
  Delay{,1..6,9} (8 alike) : Delay  DelayLength=4
  Generate Signal for End of Frame : Subsystem
  Read Offset Address Signals Generator : MATLAB Function  TreatAsAtomicUnit=on
  Terminator : Terminator
  readAddr : Outport
  readValid : Outport  Port=2
  startOut : Outport  Port=3
  endOut : Outport  Port=4
  wires:
  Delay6/1 -> startOut/1
  Read Offset Address Signals Generator/3(curRorCOut) -> Compute Read Offset Address/3(curC)
  Read Offset Address Signals Generator/2(maxRorCOut) -> Compute Read Offset Address/2(maxC)
  Read Offset Address Signals Generator/1(curCorROut) -> Compute Read Offset Address/1(curR)
  Compute Read Offset Address/1(addr) -> readAddr/1
  Read Offset Address Signals Generator/4(modcodIs12Out) -> Terminator/1
  Delay9/1 -> readValid/1
  Delay5/1 -> endOut/1
  Delay4/1 -> Read Offset Address Signals Generator/6(wrEnb)
  Delay3/1 -> Read Offset Address Signals Generator/5(wrAddr)
  Delay2/1 -> Read Offset Address Signals Generator/4(modcodIs12)
  Delay1/1 -> Read Offset Address Signals Generator/3(maxC)
  Delay/1 -> Read Offset Address Signals Generator/1(maxR)
  Generate Signal for End of Frame/1(chkwrAddrEnd) -> Read Offset Address Signals Generator/2(chkwrAddrEnd)
  maxR/1 -> Delay/1, Generate Signal for End of Frame/1(maxR)
  maxC/1 -> Delay1/1, Generate Signal for End of Frame/2(maxC)
  Read Offset Address Signals Generator/6(endOut) -> Delay5/1
  Read Offset Address Signals Generator/5(startOut) -> Delay6/1
  Read Offset Address Signals Generator/7(readValid) -> Delay9/1
  wrEnb/1 -> Delay4/1
  wrAddr/1 -> Delay3/1
  modcodIs12/1 -> Delay2/1

== system soc_dvbs2_fpga/DVBS2/DVBS2 TxRx/DVB-S2 HDL Receiver/Demod Deinterleave and FECDecode/DVBS2 HDL Deinterleaver/RAM Address Generator/Write Offset Address ==
  fecframe : Inport
  enb : Inport  Port=2
  Compare To Constant : simulink/Logic and Bit Operations/Compare To Constant  relop===  const=ConfigRx.ShortFrameLen - 1  OutDataTypeStr=boolean
  Data Type Duplicate : DataTypeDuplicate
  Data Type Conversion : DataTypeConversion  SaturateOnIntegerOverflow=off  RndMeth=Floor
  Delay{1..12} (12 alike) : Delay  DelayLength=1
  Logical Operator : Logic  Inputs=3  AllPortsSameDT=off  OutDataTypeStr=boolean
  Switch : Switch  Criteria=u2 ~= 0  SaturateOnIntegerOverflow=off  InputSameDT=off
  Write Offset Address Normal Frame : hdlsllib/Sources/HDL Counter  CountType=Count limited  CountInit=0  CountStep=1  CountMax=ConfigRx.NormalFrameLen - 1  CountFromType=Initial value  CountFrom=0  CountResetPort=on  CountLoadPort=off  CountEnbPort=on  CountDirPort=off  CountHitOutputPort=off  CountDataType=Unsigned  CountWordLen=nextpow2(ConfigRx.NormalFrameLen - 1)  CountFracLen=0  CountSampTime=1
  Write Offset Address Short Frame : hdlsllib/Sources/HDL Counter  CountType=Count limited  CountInit=0  CountStep=1  CountMax=ConfigRx.ShortFrameLen - 1  CountFromType=Initial value  CountFrom=0  CountResetPort=off  CountLoadPort=off  CountEnbPort=on  CountDirPort=off  CountHitOutputPort=off  CountDataType=Unsigned  CountWordLen=nextpow2(ConfigRx.ShortFrameLen - 1)  CountFracLen=0  CountSampTime=1
  addr : Outport
  wires:
  Delay12/1 -> Delay11/1
  fecframe/1 -> Delay12/1
  Delay10/1 -> Delay9/1, Write Offset Address Short Frame/1
  Delay9/1 -> Logical Operator/3, Delay7/1
  Delay8/1 -> Compare To Constant/1, Delay3/1
  Delay7/1 -> Write Offset Address Normal Frame/2
  Delay6/1 -> Write Offset Address Normal Frame/1
  Delay4/1 -> Delay1/1
  Delay3/1 -> Data Type Conversion/1
  Delay2/1 -> Switch/3
  Delay1/1 -> Switch/2
  Delay5/1 -> Switch/1
  Data Type Conversion/1 -> Data Type Duplicate/1, Delay5/1
  Delay11/1 -> Delay4/1, Logical Operator/1
  Logical Operator/1 -> Delay6/1
  Switch/1 -> addr/1
  Compare To Constant/1 -> Logical Operator/2
  Write Offset Address Short Frame/1 -> Delay8/1
  Write Offset Address Normal Frame/1 -> Data Type Duplicate/2, Delay2/1
  enb/1 -> Delay10/1

== system soc_dvbs2_fpga/DVBS2/DVBS2 TxRx/DVB-S2 HDL Receiver/Demod Deinterleave and FECDecode/DVBS2 HDL Deinterleaver/RAM Address Generator/nRows and nColumns ==
  captureIn : Inport
  modIdx : Inport  Port=2
  codIdx : Inport  Port=3
  fecFrame : Inport  Port=4
  Compare To Constant : simulink/Logic and Bit Operations/Compare To Constant  relop===  const=1  OutDataTypeStr=boolean
  Compare To Constant1 : simulink/Logic and Bit Operations/Compare To Constant  relop===  const=4  OutDataTypeStr=boolean
  Data Type Duplicate : DataTypeDuplicate
  Data Type Conversion : DataTypeConversion  SaturateOnIntegerOverflow=off  RndMeth=Floor
  Delay{1..14} (14 alike) : Delay
  Logical Operator : Logic  AllPortsSameDT=off  OutDataTypeStr=boolean
  MaxC LUT : Lookup_n-D  NumberOfTableDimensions=1  BreakpointsSpecification=Even spacing  BreakpointsForDimension1=[-5:5]  BreakpointsForDimension1FirstPoint=0  Table=[1 3 4 5]  TableDataTypeStr=fixdt(0,3,0)  InterpMethod=Flat  InternalRulePriority=Speed  OutDataTypeStr=fixdt(0,3,0)  RndMeth=Simplest
  MaxR Normal LUT : Lookup_n-D  NumberOfTableDimensions=1  BreakpointsSpecification=Even spacing  BreakpointsForDimension1=[-5:5]  BreakpointsForDimension1FirstPoint=0  Table=64800./[1 3 4 5]  TableDataTypeStr=fixdt(0,nextpow2(64800),0)  InterpMethod=Flat  InternalRulePriority=Speed  OutDataTypeStr=fixdt(0,nextpow2(64800),0)  RndMeth=Simplest
  MaxR Short LUT : Lookup_n-D  NumberOfTableDimensions=1  BreakpointsSpecification=Even spacing  BreakpointsForDimension1=[-5:5]  BreakpointsForDimension1FirstPoint=0  Table=16200./[1 3 4 5]  TableDataTypeStr=fixdt(0,nextpow2(16200),0)  InterpMethod=Flat  InternalRulePriority=Speed  OutDataTypeStr=fixdt(0,nextpow2(16200),0)  RndMeth=Simplest
  maxR_switch : MultiPortSwitch  DataPortOrder=Zero-based contiguous  Inputs=2  zeroidx=on  SaturateOnIntegerOverflow=off  InputSameDT=off
  captureOut : Outport
  modIdxOut : Outport  Port=2
  codIdxOut : Outport  Port=3
  fecFrameOut : Outport  Port=4
  maxR : Outport  Port=5
  maxC : Outport  Port=6
  isMODOCD12 : Outport  Port=7
  wires:
  Delay14/1 -> maxR_switch/2, Data Type Duplicate/1
  Delay13/1 -> Data Type Conversion/1
  Delay12/1 -> maxC/1
  Delay11/1 -> MaxC LUT/1
  Delay10/1 -> MaxR Short LUT/1
  Delay9/1 -> MaxR Normal LUT/1
  Delay8/1 -> Compare To Constant1/1, codIdxOut/1
  Delay7/1 -> Compare To Constant/1, modIdxOut/1
  Delay6/1 -> Delay8/1
  Delay5/1 -> Delay7/1
  Delay4/1 -> captureOut/1
  Delay3/1 -> maxR_switch/1, fecFrameOut/1
  Delay2/1 -> Delay4/1
  Delay1/1 -> Delay3/1
  captureIn/1 -> Delay2/1
  Compare To Constant/1 -> Logical Operator/1
  codIdx/1 -> Delay6/1
  Logical Operator/1 -> isMODOCD12/1
  Compare To Constant1/1 -> Logical Operator/2
  modIdx/1 -> Delay9/1, Delay10/1, Delay11/1, Delay5/1
  maxR_switch/1 -> maxR/1
  MaxC LUT/1 -> Delay12/1
  fecFrame/1 -> Delay1/1
  MaxR Short LUT/1 -> Delay13/1
  Data Type Conversion/1 -> maxR_switch/3, Data Type Duplicate/2
  MaxR Normal LUT/1 -> Delay14/1

== system soc_dvbs2_fpga/DVBS2/DVBS2 TxRx/DVB-S2 HDL Receiver/Stream Recovery/BB Decoder/Extract BBHeader/Extract DFL ==
  bitsIn : Inport
  idx : Inport  Port=2
  validIn : Inport  Port=3
  Add : Sum  Inputs=|++  OutDataTypeStr=Inherit: Same as first input
  Compare To Constant : simulink/Logic and Bit Operations/Compare To Constant  relop=>=  const=32  OutDataTypeStr=boolean
  Compare To Constant1 : simulink/Logic and Bit Operations/Compare To Constant  relop=<=  const=32+15  OutDataTypeStr=boolean
  Compare To Constant2 : simulink/Logic and Bit Operations/Compare To Constant  relop===  const=48  OutDataTypeStr=boolean
  Data Type Conversion : DataTypeConversion  OutDataTypeStr=uint16  SaturateOnIntegerOverflow=off  RndMeth=Floor
  Gain : Gain  Gain=2  ParamDataTypeStr=fixdt(0,2,0)  OutDataTypeStr=Inherit: Same as input
  Logical Operator : Logic  Inputs=3  AllPortsSameDT=off  OutDataTypeStr=boolean
  Logical Operator1 : Logic  AllPortsSameDT=off  OutDataTypeStr=boolean
  Unit Delay Enabled Synchronous : hdlsllib/Discrete/Unit Delay Enabled Synchronous  InitialCondition=0.0  SampleTime=-1
  Unit Delay Enabled Resettable Synchronous : hdlsllib/Discrete/Unit Delay Enabled Resettable Synchronous  InitialCondition=0.0  SampleTime=-1
  DFL : Outport
  wires:
  bitsIn/1 -> Data Type Conversion/1
  Compare To Constant1/1 -> Logical Operator/2
  Gain/1 -> Add/2
  Unit Delay Enabled Synchronous/1 -> DFL/1
  Data Type Conversion/1 -> Add/1
  Compare To Constant2/1 -> Logical Operator1/1
  Unit Delay Enabled Resettable Synchronous/1 -> Unit Delay Enabled Synchronous/1, Gain/1
  idx/1 -> Compare To Constant/1, Compare To Constant1/1, Compare To Constant2/1
  Add/1 -> Unit Delay Enabled Resettable Synchronous/1
  Logical Operator/1 -> Unit Delay Enabled Resettable Synchronous/2
  validIn/1 -> Logical Operator/3, Logical Operator1/2
  Logical Operator1/1 -> Unit Delay Enabled Resettable Synchronous/3, Unit Delay Enabled Synchronous/2
  Compare To Constant/1 -> Logical Operator/1
